simulink model "direct_graph_2D_spanning_tree"  (R2020a)
settings: Solver=FixedStepAuto  StartTime=0.0  StopTime=10.0  FixedStep=0.0001  RelTol=1e-3
libraries: fod x2
settings Model: Creator=WangQipeng  LastModifiedBy=WangQipeng

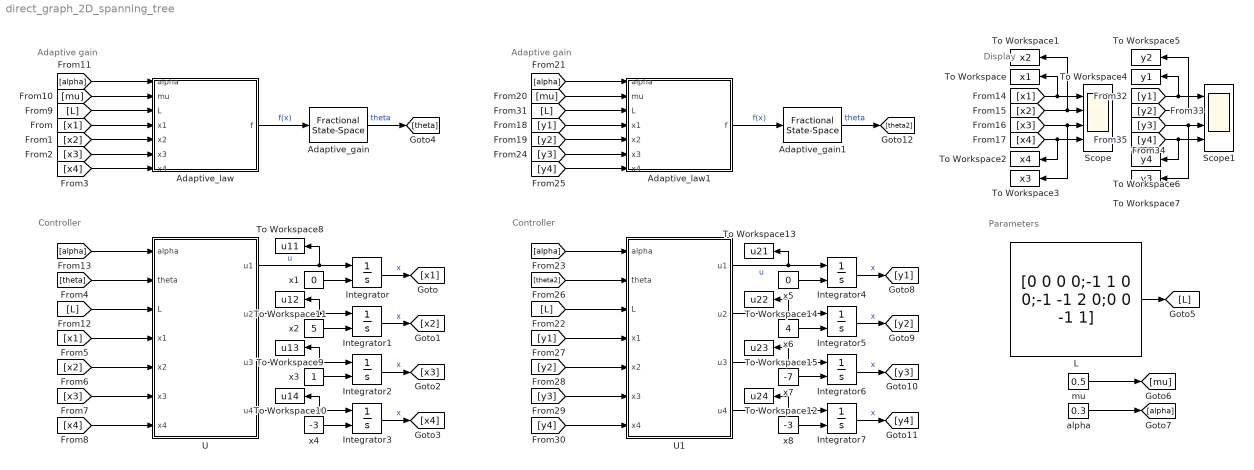
== system direct_graph_2D_spanning_tree ==
  note: Controller
  note: Adaptive gain
  note: Display
  note: Parameters
  note: Controller
  note: Adaptive gain
  Adaptive_gain : fod/Fractional State-Space  A=0  B=1  C=1  D=0  q=0.5  iniOff=[0]  freqRange=[0.0001 10000]  approxNum=5  useRef=off  mask(FOSS){}
      settings: SourceProductName=FOMCON Toolbox
      mask Display: disp(['D^\beta \theta=f(x)'], 'TeXMode', 'On');
  Adaptive_gain1 : fod/Fractional State-Space  A=0  B=1  C=1  D=0  q=0.5  iniOff=[0]  freqRange=[0.0001 10000]  approxNum=5  useRef=off  mask(FOSS){}
      settings: SourceProductName=FOMCON Toolbox
      mask Display: disp(['D^\beta \theta=f(x)'], 'TeXMode', 'On');
  Adaptive_law : MATLAB Function  TreatAsAtomicUnit=on
  Adaptive_law1 : MATLAB Function  TreatAsAtomicUnit=on
  Integrator{,1..7} (8 alike) : Integrator  InitialConditionSource=external  InitialCondition=1
  L : Constant  Value=[0 0 0 0;-1 1 0 0;-1 -1 2 0;0 0 -1 1]
  Scope : Scope  NumInputPorts=4
  Scope1 : Scope  NumInputPorts=4
  To Workspace : ToWorkspace  VariableName=x1  SaveFormat=Timeseries  SampleTime=-1
  To Workspace1 : ToWorkspace  VariableName=x2  SaveFormat=Timeseries  SampleTime=-1
  To Workspace10 : ToWorkspace  VariableName=u14  SaveFormat=Timeseries  SampleTime=-1
  To Workspace11 : ToWorkspace  VariableName=u12  SaveFormat=Timeseries  SampleTime=-1
  To Workspace12 : ToWorkspace  VariableName=u24  SaveFormat=Timeseries  SampleTime=-1
  To Workspace13 : ToWorkspace  VariableName=u21  SaveFormat=Timeseries  SampleTime=-1
  To Workspace14 : ToWorkspace  VariableName=u22  SaveFormat=Timeseries  SampleTime=-1
  To Workspace15 : ToWorkspace  VariableName=u23  SaveFormat=Timeseries  SampleTime=-1
  To Workspace2 : ToWorkspace  VariableName=x4  SaveFormat=Timeseries  SampleTime=-1
  To Workspace3 : ToWorkspace  VariableName=x3  SaveFormat=Timeseries  SampleTime=-1
  To Workspace4 : ToWorkspace  VariableName=y1  SaveFormat=Timeseries  SampleTime=-1
  To Workspace5 : ToWorkspace  VariableName=y2  SaveFormat=Timeseries  SampleTime=-1
  To Workspace6 : ToWorkspace  VariableName=y4  SaveFormat=Timeseries  SampleTime=-1
  To Workspace7 : ToWorkspace  VariableName=y3  SaveFormat=Timeseries  SampleTime=-1
  To Workspace8 : ToWorkspace  VariableName=u11  SaveFormat=Timeseries  SampleTime=-1
  To Workspace9 : ToWorkspace  VariableName=u13  SaveFormat=Timeseries  SampleTime=-1
  U : MATLAB Function  TreatAsAtomicUnit=on
  U1 : MATLAB Function  TreatAsAtomicUnit=on
  alpha : Constant  Value=0.3
  mu : Constant  Value=0.5
  x1 : Constant  Value=0
  x2 : Constant  Value=5
  x3 : Constant
  x4 : Constant  Value=-3
  x5 : Constant  Value=0
  x6 : Constant  Value=4
  x7 : Constant  Value=-7
  x8 : Constant  Value=-3
  wires:
  U/1(u1) -> To Workspace8/1, Integrator/1  "u"
  Adaptive_law/1(f) -> Adaptive_gain/1  "f(x)"
  U/2(u2) -> To Workspace11/1, Integrator1/1
  U/3(u3) -> To Workspace9/1, Integrator2/1
  U/4(u4) -> To Workspace10/1, Integrator3/1
  Integrator/1 -> [x1]  "x"
  [x1] -> Adaptive_law/4(x1)
  Integrator1/1 -> [x2]  "x"
  Integrator2/1 -> [x3]  "x"
  Integrator3/1 -> [x4]  "x"
  [x2] -> Adaptive_law/5(x2)
  [x3] -> Adaptive_law/6(x3)
  [x4] -> Adaptive_law/7(x4)
  Adaptive_gain/1 -> [theta]  "theta"
  [theta] -> U/2(theta)
  [x3] -> U/6(x3)
  [x4] -> U/7(x4)
  [x1] -> U/4(x1)
  [x2] -> U/5(x2)
  L/1 -> [L]
  [L] -> Adaptive_law/3(L)
  mu/1 -> [mu]
  alpha/1 -> [alpha]
  [mu] -> Adaptive_law/2(mu)
  [alpha] -> Adaptive_law/1(alpha)
  [L] -> U/3(L)
  [alpha] -> U/1(alpha)
  x1/1 -> Integrator/2
  x2/1 -> Integrator1/2
  x3/1 -> Integrator2/2
  x4/1 -> Integrator3/2
  [x1] -> Scope/1, To Workspace/1
  [x2] -> To Workspace1/1, Scope/2
  [x3] -> Scope/3, To Workspace3/1
  [x4] -> Scope/4, To Workspace2/1
  Integrator6/1 -> [y3]  "x"
  [y4] -> Adaptive_law1/7(x4)
  [alpha] -> U1/1(alpha)
  Integrator5/1 -> [y2]  "x"
  U1/3(u3) -> To Workspace15/1, Integrator6/1
  [y3] -> Adaptive_law1/6(x3)
  U1/2(u2) -> To Workspace14/1, Integrator5/1
  U1/4(u4) -> To Workspace12/1, Integrator7/1
  x6/1 -> Integrator5/2
  x5/1 -> Integrator4/2
  [mu] -> Adaptive_law1/2(mu)
  [alpha] -> Adaptive_law1/1(alpha)
  [L] -> U1/3(L)
  [y1] -> U1/4(x1)
  Adaptive_law1/1(f) -> Adaptive_gain1/1  "f(x)"
  U1/1(u1) -> To Workspace13/1, Integrator4/1  "u"
  [y4] -> U1/7(x4)
  [theta2] -> U1/2(theta)
  Adaptive_gain1/1 -> [theta2]  "theta"
  x7/1 -> Integrator6/2
  [L] -> Adaptive_law1/3(L)
  [y1] -> Adaptive_law1/4(x1)
  [y2] -> Adaptive_law1/5(x2)
  [y3] -> U1/6(x3)
  Integrator4/1 -> [y1]  "x"
  Integrator7/1 -> [y4]  "x"
  [y2] -> U1/5(x2)
  x8/1 -> Integrator7/2
  [y1] -> Scope1/1, To Workspace4/1
  [y3] -> Scope1/3, To Workspace7/1
  [y4] -> Scope1/4, To Workspace6/1
  [y2] -> To Workspace5/1, Scope1/2

== matlab function direct_graph_2D_spanning_tree/U ==
  data: alpha input; u1 output; theta input; L input; x1 input; x2 input; x3 input; x4 input; u2 output; u3 output; u4 output
function [u1,u2,u3,u4] = protocol(alpha,theta,L,x1,x2,x3,x4)
x = [x1;x2;x3;x4];
temp = -L * x;
%temp_u1 = temp(1);
temp_u2 = temp(2);
temp_u3 = temp(3);
temp_u4 = temp(4);


u1 = 0;
u2 = theta * sign(temp_u2) * abs(temp_u2)^(alpha);
u3 = theta * sign(temp_u3) * abs(temp_u3)^(alpha);
u4 = theta * sign(temp_u4) * abs(temp_u4)^(alpha);

== matlab function direct_graph_2D_spanning_tree/Adaptive_law ==
  data: alpha input; f output; mu input; L input; x1 input; x2 input; x3 input; x4 input
function f = Lyapunov_Like(alpha,mu,L,x1,x2,x3,x4)
% h = [2;1;1];
x = [x1;x2;x3;x4];
% L = [  0      0      0       0;
%         -1     1      0       0;
%         -1    -1      2       0;
%         0      0      -1      1];

P_L = 2/(1+alpha) * abs(L(2,:)*x)^(1+alpha) ...
      + 1/(1+alpha) * abs(L(3,:)*x)^(1+alpha) ...
      + 2/(1+alpha) * abs(L(4,:)*x)^(1+alpha);
f = mu * abs(P_L)^((1-alpha)/(1+alpha));

== matlab function direct_graph_2D_spanning_tree/Adaptive_law1 ==
  data: alpha input; f output; mu input; L input; x1 input; x2 input; x3 input; x4 input
function f = Lyapunov_Like(alpha,mu,L,x1,x2,x3,x4)
% h = [2;1;1];
x = [x1;x2;x3;x4];
% L = [  0      0      0       0;
%         -1     1      0       0;
%         -1    -1      2       0;
%         0      0      -1      1];

P_L = 2/(1+alpha) * abs(L(2,:)*x)^(1+alpha) ...
      + 1/(1+alpha) * abs(L(3,:)*x)^(1+alpha) ...
      + 2/(1+alpha) * abs(L(4,:)*x)^(1+alpha);
f = mu * abs(P_L)^((1-alpha)/(1+alpha));

== matlab function direct_graph_2D_spanning_tree/U1 ==
  data: alpha input; u1 output; theta input; L input; x1 input; x2 input; x3 input; x4 input; u2 output; u3 output; u4 output
function [u1,u2,u3,u4] = protocol(alpha,theta,L,x1,x2,x3,x4)
x = [x1;x2;x3;x4];
temp = -L * x;
%temp_u1 = temp(1);
temp_u2 = temp(2);
temp_u3 = temp(3);
temp_u4 = temp(4);


u1 = 0;
u2 = theta * sign(temp_u2) * abs(temp_u2)^(alpha);
u3 = theta * sign(temp_u3) * abs(temp_u3)^(alpha);
u4 = theta * sign(temp_u4) * abs(temp_u4)^(alpha);
